simulink model "L9_Realisation_digital_filters"  (R2023b)
settings: Solver=VariableStepAuto  StartTime=0.0  StopTime=10.0  RelTol=1e-3
settings Model: Creator=patel
settings SolverCC: AlgebraicLoopSolver=TrustRegion
settings DebuggingCC: UnconnectedInputMsg=warning  UnconnectedOutputMsg=warning  UnconnectedLineMsg=warning
settings ModelReferenceCC: EnableRefExpFcnMdlSchedulingChecks=on

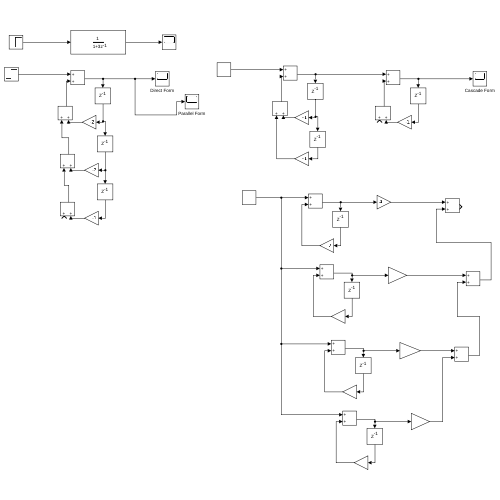
[thumbnail: Simulink's stored preview of the top-level diagram]
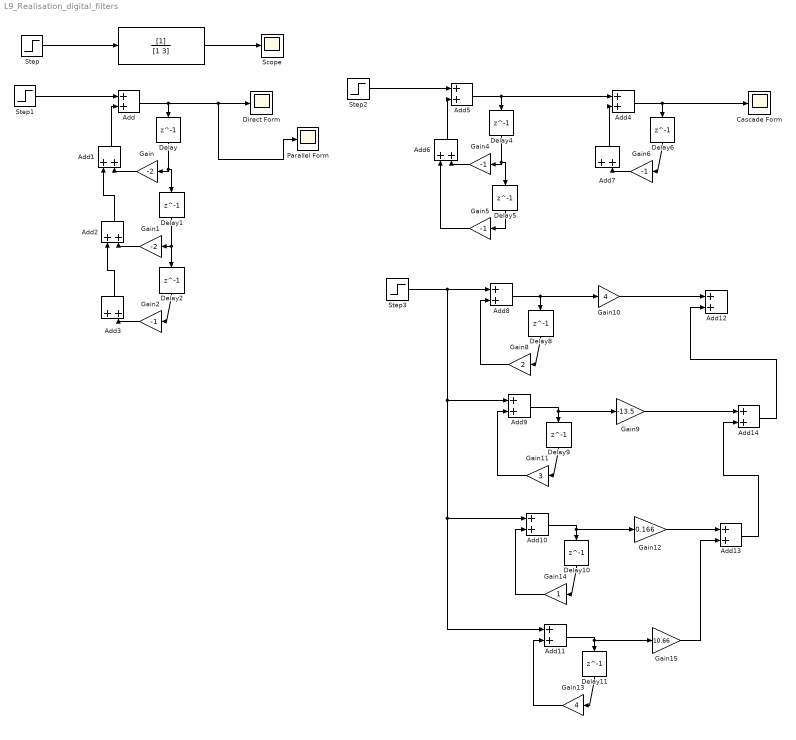
== system L9_Realisation_digital_filters ==
  " " : DiscreteFilter  Denominator=[1 3]
  Add{,1..14} (15 alike) : Sum
  "Cascade Form " : Scope
  Delay{,1..2,4..6,8..11} (10 alike) : Delay  DelayLength=1
  "Direct Form " : Scope
  Gain : Gain  Gain=-2
  Gain1 : Gain  Gain=-2
  Gain10 : Gain  Gain=4
  Gain11 : Gain  Gain=3
  Gain12 : Gain  Gain=0.166
  Gain13 : Gain  Gain=4
  Gain14 : Gain
  Gain15 : Gain  Gain=10.66
  Gain{2,4..6} (4 alike) : Gain  Gain=-1
  Gain8 : Gain  Gain=2
  Gain9 : Gain  Gain=-13.5
  Parallel Form : Scope
  Scope : Scope
  Step{,1..3} (4 alike) : Step  SampleTime=0
  wires:
  Step/1 -> " "/1
  " "/1 -> Scope/1
  Step1/1 -> Add/1
  Delay/1 -> Delay1/1, Gain/1
  Gain/1 -> Add1/2
  Gain1/1 -> Add2/2
  Delay1/1 -> Delay2/1, Gain1/1
  Add2/1 -> Add1/1
  Gain2/1 -> Add3/2
  Delay2/1 -> Gain2/1
  Add3/1 -> Add2/1
  Add1/1 -> Add/2
  Add6/1 -> Add5/2
  Gain5/1 -> Add6/1
  Add5/1 -> Add4/1, Delay4/1
  Delay4/1 -> Delay5/1, Gain4/1
  Step2/1 -> Add5/1
  Gain4/1 -> Add6/2
  Delay5/1 -> Gain5/1
  Add7/1 -> Add4/2
  Add4/1 -> "Cascade Form "/1, Delay6/1
  Delay6/1 -> Gain6/1
  Gain6/1 -> Add7/2
  Gain8/1 -> Add8/2
  Add8/1 -> Gain10/1, Delay8/1
  Delay8/1 -> Gain8/1
  Gain11/1 -> Add9/2
  Delay9/1 -> Gain11/1
  Add9/1 -> Gain9/1, Delay9/1
  Gain14/1 -> Add10/2
  Delay10/1 -> Gain14/1
  Step3/1 -> Add9/1, Add10/1, Add11/1, Add8/1
  Delay11/1 -> Gain13/1
  Gain13/1 -> Add11/2
  Add11/1 -> Gain15/1, Delay11/1
  Add10/1 -> Gain12/1, Delay10/1
  Gain10/1 -> Add12/1
  Gain12/1 -> Add13/1
  Gain15/1 -> Add13/2
  Add13/1 -> Add14/2
  Gain9/1 -> Add14/1
  Add14/1 -> Add12/2
  Add/1 -> Delay/1, Parallel Form/1, "Direct Form "/1
